simulink model "Kiwi_control"  (R2014a)
settings: Solver=FixedStepDiscrete  StartTime=0.0  StopTime=inf  FixedStep=0.008  RelTol=1e-3
undefined symbols (not defined in the file or in its folder): Encoder_counts, Kr, Krq, Prijenosni_omjeri, Ti, Ts, Ucc
libraries: simulink_extras x4, simulink x1
settings Model: SimulationMode=external  Creator=damir  LastModifiedBy=ante
settings SolverCC: AutoInsertRateTranBlk=on
settings DataIOCC: LimitDataPoints=off
settings OptimizationCC: OptimizeModelRefInitCode=on  LifeSpan=1
settings RTWCC: SystemTargetFile=ert_linux.tlc  TemplateMakefile=ert_linux.tmf  Description=Linux Embedded Coder  ProcessScript=ert_linux_make_rtw_hook  BuildConfiguration=Specify
settings RTWCC: CustomSource=|
  | bci.c
  | ipci.c
  | pc_i.c
  | bapfw165.c
  | filterlist.c
  | bapfw320.c
  | ipci_lin.c
  | bapfw161.c
  | dpram.c
  | kiwi.c
settings CodeAppCC: IgnoreCustomStorageClasses=off
settings STFCustomTargetCC: CodeReplacementLibrary=GNU C99 extensions  ModelReferenceCompliant=off  ConcurrentExecutionCompliant=off  GeneratePreprocessorConditionals=Use local settings  CombineOutputUpdateFcns=on  ERTCustomFileBanners=on  MATLABClassNameForMDSCustomization=Simulink.SoftwareTarget.ERTCustomization  GRTInterface=off  SystemTargetFile=ert_linux.tlc
settings ERTTargetCC: CodeReplacementLibrary=GNU C99 extensions  GenerateSampleERTMain=off  ModelReferenceCompliant=off  SupportContinuousTime=on  SupportNonInlinedSFcns=on  ExtMode=on  ExtModeMexArgs='161.53.68.185' 1 17725  ERTCustomFileTemplate=ert_linux_file_process.tlc

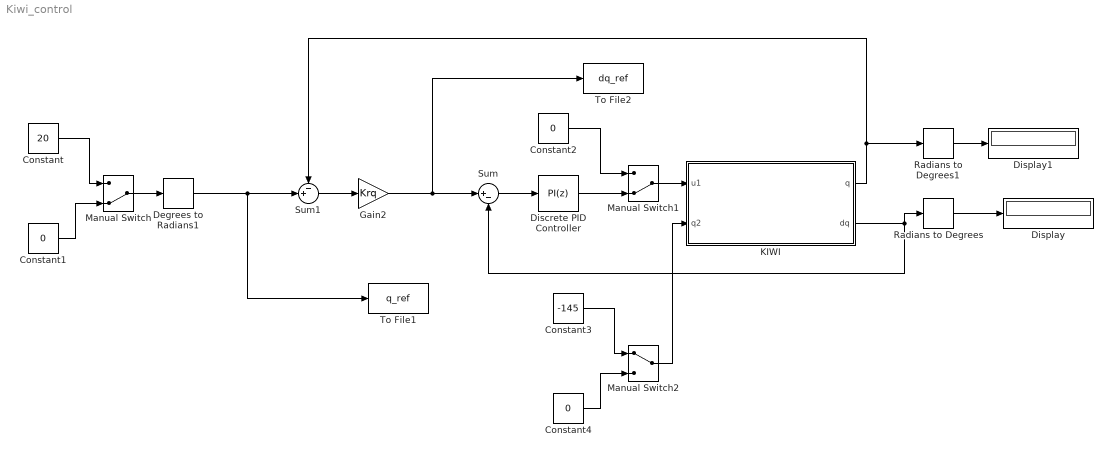
== system Kiwi_control ==
  Constant : Constant  Value=20
  Constant1 : Constant  Value=0
  Constant2 : Constant  Value=0
  Constant3 : Constant  Value=-145
  Constant4 : Constant  Value=0
  Degrees to Radians1 : simulink_extras/Transformations/Degrees to Radians
  Discrete PID Controller : simulink/Continuous/PID Controller  Controller=PI  TimeDomain=Discrete-time  SampleTime=Ts  IntegratorMethod=Forward Euler  FilterMethod=Forward Euler  Form=Parallel  P=Kr  I=Kr/Ti  D=0  N=100  InitialConditionSource=internal  InitialConditionForIntegrator=0  InitialConditionForFilter=0  ExternalReset=none  LimitOutput=on  UpperSaturationLimit=24  LowerSaturationLimit=-24  LinearizeAsGain=off  AntiWindupMode=clamping  Kb=1  TrackingMode=off  Kt=1  PParamMin=[]  PParamMax=[]  IParamMin=[]  IParamMax=[]  DParamMin=[]  DParamMax=[]  NParamMin=[]  NParamMax=[]  KbParamMin=[]  KbParamMax=[]  KtParamMin=[]  KtParamMax=[]  POutMin=[]  POutMax=[]  IOutMin=[]  IOutMax=[]  DOutMin=[]  DOutMax=[]  NOutMin=[]  NOutMax=[]  KbOutMin=[]  KbOutMax=[]  KtOutMin=[]  KtOutMax=[]  IntegratorOutMin=[]  IntegratorOutMax=[]  FilterOutMin=[]  FilterOutMax=[]  SumOutMin=[]  SumOutMax=[]  SumI1OutMin=[]  SumI1OutMax=[]  SumI2OutMin=[]  SumI2OutMax=[]  SumI3OutMin=[]  SumI3OutMax=[]  SumDOutMin=[]  SumDOutMax=[]  SaturationOutMin=[]  SaturationOutMax=[]  IntegratorContinuousStateAttributes=''  IntegratorStateMustResolveToSignalObject=off  IntegratorRTWStateStorageClass=Auto  FilterContinuousStateAttributes=''  FilterStateMustResolveToSignalObject=off  FilterRTWStateStorageClass=Auto
  Display : Display
  Display1 : Display
  Gain2 : Gain  Gain=Krq
  KIWI : Subsystem
  Manual Switch : ManualSwitch  CurrentSetting=0
  Manual Switch1 : ManualSwitch  CurrentSetting=0
  Manual Switch2 : ManualSwitch
  Radians to Degrees : simulink_extras/Transformations/Radians to Degrees
  Radians to Degrees1 : simulink_extras/Transformations/Radians to Degrees
  Sum : Sum  Inputs=|+-
  Sum1 : Sum  Inputs=-+|
  To File1 : ToFile  Filename=q_ref  MatrixName=q_ref  SampleTime=Ts
  To File2 : ToFile  Filename=dq_ref  MatrixName=dq_ref  SampleTime=Ts
  wires:
  Constant/1 -> Manual Switch/1
  Constant1/1 -> Manual Switch/2
  Sum/1 -> Discrete PID Controller/1
  KIWI/2(dq) -> Radians to Degrees/1, Sum/2
  KIWI/1(q) -> Sum1/1, Radians to Degrees1/1
  Radians to Degrees/1 -> Display/1
  Radians to Degrees1/1 -> Display1/1
  Manual Switch1/1 -> KIWI/1(u1)
  Constant2/1 -> Manual Switch1/1
  Manual Switch/1 -> Degrees to Radians1/1
  Sum1/1 -> Gain2/1
  Constant3/1 -> Manual Switch2/1
  Constant4/1 -> Manual Switch2/2
  Manual Switch2/1 -> KIWI/2(q2)
  Discrete PID Controller/1 -> Manual Switch1/2
  Degrees to Radians1/1 -> Sum1/2, To File1/1
  Gain2/1 -> To File2/1, Sum/1

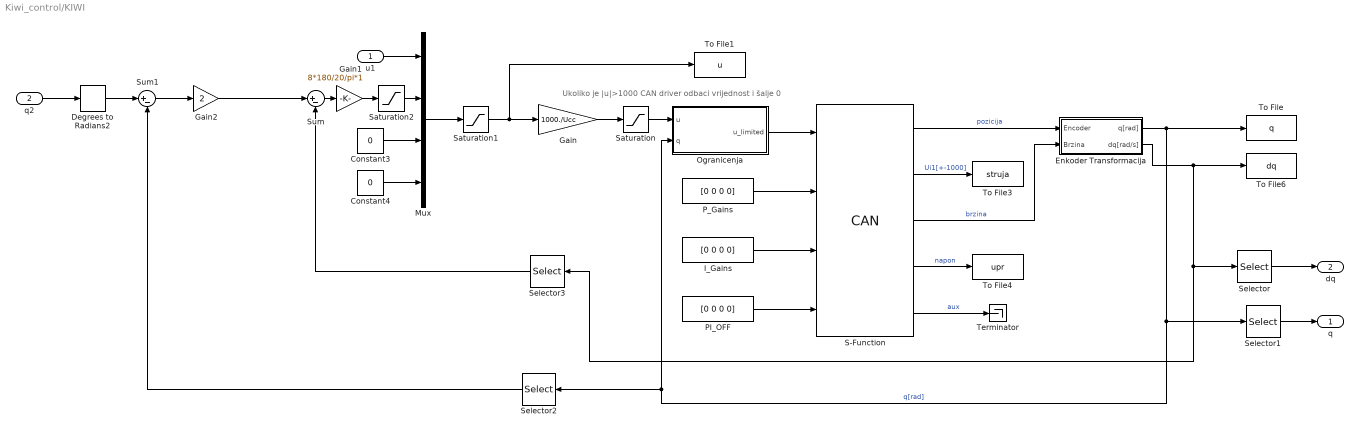
== system Kiwi_control/KIWI ==
  note: Ukoliko je |u|>1000 CAN driver odbaci vrijednost i šalje 0
  u1 : Inport
  q2 : Inport  Port=2
  Constant3 : Constant  Value=0
  Constant4 : Constant  Value=0
  Degrees to Radians2 : simulink_extras/Transformations/Degrees to Radians
  Enkoder Transformacija : Subsystem
  Gain : Gain  Gain=1000./Ucc
  Gain1 : Gain  Gain=8*180/20/pi*1
  Gain2 : Gain  Gain=2
  I_Gains : Constant  Value=[0 0 0 0]
  Mux : Mux
  Ogranicenja : MATLAB Function  TreatAsAtomicUnit=on
  PI_OFF : Constant  Value=[0 0 0 0]
  P_Gains : Constant  Value=[0 0 0 0]
  S-Function : S-Function  FunctionName=CAN  EnableBusSupport=off
  Saturation : Saturate  UpperLimit=+1000  LowerLimit=-1000
  Saturation1 : Saturate  UpperLimit=24  LowerLimit=-24
  Saturation2 : Saturate  UpperLimit=8  LowerLimit=-8
  Selector : Selector  InputPortWidth=4
  Selector1 : Selector  InputPortWidth=4
  Selector2 : Selector  InputPortWidth=4  Indices=2
  Selector3 : Selector  InputPortWidth=4  Indices=2
  Sum : Sum  Inputs=|+-
  Sum1 : Sum  Inputs=|+-
  Terminator : Terminator
  To File : ToFile  Filename=q  MatrixName=q
  To File1 : ToFile  Filename=u  MatrixName=u  SampleTime=Ts
  To File3 : ToFile  Filename=struja  MatrixName=struja  SampleTime=Ts
  To File4 : ToFile  Filename=upr  MatrixName=upr  SampleTime=Ts
  To File6 : ToFile  Filename=dq  MatrixName=dq
  q : Outport
  dq : Outport  Port=2
  wires:
  Mux/1 -> Saturation1/1
  I_Gains/1 -> S-Function/3
  Gain1/1 -> Saturation2/1
  P_Gains/1 -> S-Function/2
  Enkoder Transformacija/2(dq[rad/s]) -> Selector3/1, Selector/1, To File6/1
  S-Function/3 -> Enkoder Transformacija/2(Brzina)  "brzina"
  S-Function/1 -> Enkoder Transformacija/1(Encoder)  "pozicija"
  Constant3/1 -> Mux/3
  S-Function/4 -> To File4/1  "napon"
  Constant4/1 -> Mux/4
  Enkoder Transformacija/1(q[rad]) -> Ogranicenja/2(q), Selector2/1, Selector1/1, To File/1  "q[rad]"
  S-Function/5 -> Terminator/1  "aux"
  PI_OFF/1 -> S-Function/4
  Gain/1 -> Saturation/1
  S-Function/2 -> To File3/1  "Ui1[+-1000]"
  Ogranicenja/1(u_limited) -> S-Function/1
  u1/1 -> Mux/1
  Selector/1 -> dq/1
  Selector1/1 -> q/1
  Saturation/1 -> Ogranicenja/1(u)
  Saturation1/1 -> To File1/1, Gain/1
  Sum/1 -> Gain1/1
  Gain2/1 -> Sum/1
  Sum1/1 -> Gain2/1
  Selector3/1 -> Sum/2
  Selector2/1 -> Sum1/2
  q2/1 -> Degrees to Radians2/1
  Degrees to Radians2/1 -> Sum1/1
  Saturation2/1 -> Mux/2

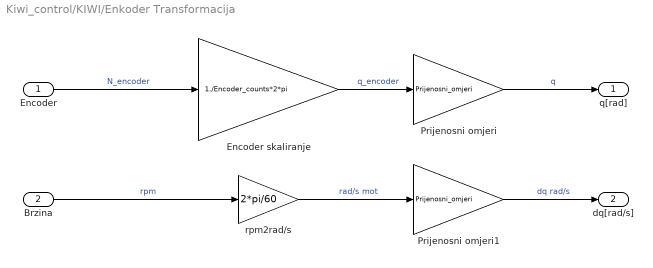
== system Kiwi_control/KIWI/Enkoder Transformacija ==
  Encoder : Inport
  Brzina : Inport  Port=2
  Encoder skaliranje : Gain  Gain=1./Encoder_counts*2*pi
  Prijenosni omjeri : Gain  Gain=Prijenosni_omjeri
  Prijenosni omjeri1 : Gain  Gain=Prijenosni_omjeri
  rpm2rad/s : Gain  Gain=2*pi/60
  q[rad] : Outport
  dq[rad/s] : Outport  Port=2
  wires:
  Encoder skaliranje/1 -> Prijenosni omjeri/1  "q_encoder"
  Prijenosni omjeri/1 -> q[rad]/1  "q"
  Encoder/1 -> Encoder skaliranje/1  "N_encoder"
  Brzina/1 -> rpm2rad/s/1  "rpm"
  rpm2rad/s/1 -> Prijenosni omjeri1/1  "rad/s mot"
  Prijenosni omjeri1/1 -> dq[rad/s]/1  "dq rad/s"

== matlab function Kiwi_control/KIWI/Ogranicenja ==
  data: u input; u_limited output; q input
function u_limited = fcn(u,q)
%#codegen
q_lim=[120,150,0,0]/180*pi;
for i=1:length(u)
 if abs(q(i))>=q_lim(i) && sign(u(i))==sign(q(i))
    u(i)=0;
 end
end

u_limited = u;
